simulink subsystem "Vehicle"  (R2023b)
settings: Solver=VariableStepAuto  StartTime=0.0  StopTime=10.0  RelTol=1e-3
undefined symbols (not defined in the file): Earth, WGS84
libraries: aerolibtransform2 x1
settings Model: Creator=szdaniel  LastModifiedBy=szdaniel

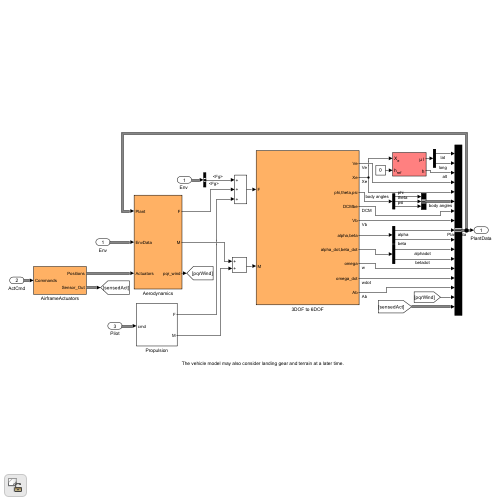
[thumbnail: Simulink's stored preview of the top-level diagram]
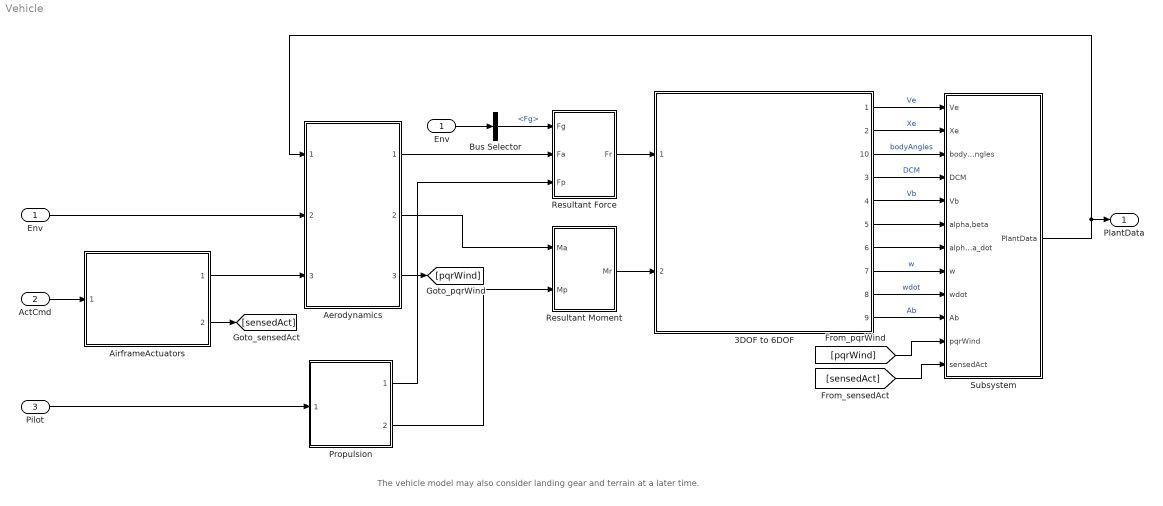
== system Vehicle ==
  note: The vehicle model may also consider landing gear and terrain at a later time.
  Env : Inport
  ActCmd : Inport  Port=2  OutDataTypeStr=Bus: ActuatorCmdBus
  Pilot : Inport  Port=3  OutDataTypeStr=Bus: PilotCmdBus
  3DOF to 6DOF : Subsystem  ReferencedSubsystem=s3DOF_to_6DOF
      settings: PortSchema="{\"entries\":[{\"content\":{\"sides\":[{\"content\":{\"connectorIds\":[\"In1\",\"In2\"]},\"type\":\"ConnectorPlacement.EquallySpacedRectSide\",\"uuid\":\"ca33f1ca-0408-408f-8b83-1949eaea45ca\"},{\"content\":{\"connectorIds\":[\"Out1\",\"Out2\",\"Out10\",\"Out3\",\"Out4\",\"Out5\",\"Out6\",\"Out7\",\"Out8\",\"Out9\"],\"side\":\"RIGHT\"},\"type\":\"ConnectorPlacement.EquallySpacedRectSide\",\"uuid\":\"ad7e90e7-3dbe-47fd-95f1-532738b13a23\"},{\"content\":{\"side\":\"TOP\"},\"type\":\"ConnectorPlacement.EquallySpacedRectSide\",\"uuid\":\"eb3caa52-9404-4bf8-ba4e-b768e3179a3f\"}]},\"type\":\"ConnectorPlacement.EquallySpacedConnector\",\"uuid\":\"d12b1c57-6f02-4c3c-8b19-49af329e35c6\"}],\"packageUris\":[\"http://schema.mathworks.com/mf0/Connector/R2020b\"],\"version\":\"1.0\"}"
  Aerodynamics : Subsystem  ReferencedSubsystem=Aerodynamics
  AirframeActuators : Subsystem  ReferencedSubsystem=AirframeActuators
  Bus Selector : BusSelector  OutputSignals=Fg
  "Env " : InportShadow
  Propulsion : Subsystem  ReferencedSubsystem=Propulsion
      settings: RTWSystemCode=Inline
  Resultant Force : Subsystem
  Resultant Moment : Subsystem
  Subsystem : Subsystem
  PlantData : Outport  VectorParamsAs1DForOutWhenUnconnected=off
  wires:
  Env/1 -> Aerodynamics/2
  ActCmd/1 -> AirframeActuators/1
  Pilot/1 -> Propulsion/1
  AirframeActuators/1 -> Aerodynamics/3
  Aerodynamics/3 -> [pqrWind]
  AirframeActuators/2 -> [sensedAct]
  Aerodynamics/2 -> Resultant Moment/1(Ma)
  Propulsion/2 -> Resultant Moment/2(Mp)
  Resultant Moment/1(Mr) -> 3DOF to 6DOF/2
  "Env "/1 -> Bus Selector/1
  Aerodynamics/1 -> Resultant Force/2(Fa)
  Propulsion/1 -> Resultant Force/3(Fp)
  Resultant Force/1(Fr) -> 3DOF to 6DOF/1
  Bus Selector/1 -> Resultant Force/1(Fg)  "<Fg>"
  Subsystem/1(PlantData) -> PlantData/1, Aerodynamics/1
  3DOF to 6DOF/1 -> Subsystem/1(Ve)  "Ve"
  3DOF to 6DOF/2 -> Subsystem/2(Xe)  "Xe"
  3DOF to 6DOF/10 -> Subsystem/3(bodyAngles)  "bodyAngles"
  3DOF to 6DOF/3 -> Subsystem/4(DCM)  "DCM"
  3DOF to 6DOF/4 -> Subsystem/5(Vb)  "Vb"
  3DOF to 6DOF/5 -> Subsystem/6(alpha,beta)
  3DOF to 6DOF/6 -> Subsystem/7(alpha_dot,beta_dot)
  3DOF to 6DOF/7 -> Subsystem/8(w)  "w"
  3DOF to 6DOF/8 -> Subsystem/9(wdot)  "wdot"
  3DOF to 6DOF/9 -> Subsystem/10(Ab)  "Ab"
  [pqrWind] -> Subsystem/11(pqrWind)
  [sensedAct] -> Subsystem/12(sensedAct)

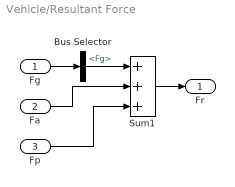
== system Vehicle/Resultant Force ==
  Fg : Inport
  Fa : Inport  Port=2
  Fp : Inport  Port=3
  Bus Selector : BusSelector  OutputSignals=Fg
  Sum1 : Sum  Inputs=+++  InputSameDT=on  SaturateOnIntegerOverflow=on  OutDataTypeStr=Inherit: Same as first input
  Fr : Outport
  wires:
  Sum1/1 -> Fr/1
  Fa/1 -> Sum1/2
  Bus Selector/1 -> Sum1/1  "<Fg>"
  Fg/1 -> Bus Selector/1
  Fp/1 -> Sum1/3

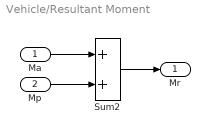
== system Vehicle/Resultant Moment ==
  Ma : Inport
  Mp : Inport  Port=2
  Sum2 : Sum  InputSameDT=on  SaturateOnIntegerOverflow=on  OutDataTypeStr=Inherit: Same as first input
  Mr : Outport
  wires:
  Sum2/1 -> Mr/1
  Ma/1 -> Sum2/1
  Mp/1 -> Sum2/2

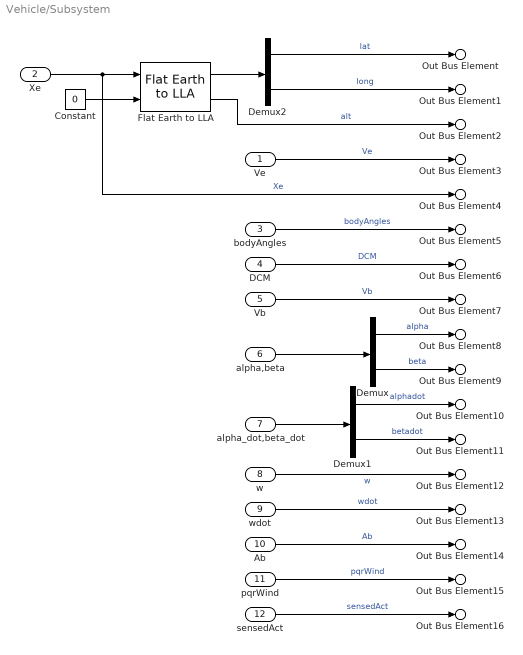
== system Vehicle/Subsystem ==
  Ve : Inport
  Xe : Inport  Port=2
  bodyAngles : Inport  Port=3
  DCM : Inport  Port=4
  Vb : Inport  Port=5
  alpha,beta : Inport  Port=6
  alpha_dot,beta_dot : Inport  Port=7
  w : Inport  Port=8
  wdot : Inport  Port=9
  Ab : Inport  Port=10
  pqrWind : Inport  Port=11
  sensedAct : Inport  Port=12
  Constant : Constant  Value=0
  Demux : Demux  Outputs=2
  Demux1 : Demux  Outputs=2
  Demux2 : Demux  Outputs=2
  Flat Earth to LLA : aerolibtransform2/Flat Earth to LLA  units=Metric (MKS)  ptype=Earth (WGS84)  F=1/298.257223563  R=6378137  refPosPort=off  LL0=LatLong0  psi=heading0
  Out Bus Element : Outport  PortName=PlantData  Element=lat
  Out Bus Element1 : Outport  PortName=PlantData  Element=lon
  Out Bus Element2 : Outport  PortName=PlantData  Element=alt
  Out Bus Element3 : Outport  PortName=PlantData  Element=Ve
  Out Bus Element4 : Outport  PortName=PlantData  Element=Xe
  Out Bus Element5 : Outport  PortName=PlantData  Element=bodyAngles
  Out Bus Element6 : Outport  PortName=PlantData  Element=DCM
  Out Bus Element7 : Outport  PortName=PlantData  Element=Vb
  Out Bus Element8 : Outport  PortName=PlantData  Element=alpha
  Out Bus Element9 : Outport  PortName=PlantData  Element=beta
  Out Bus Element10 : Outport  PortName=PlantData  Element=alphadot
  Out Bus Element11 : Outport  PortName=PlantData  Element=betadot
  Out Bus Element12 : Outport  PortName=PlantData  Element=w
  Out Bus Element13 : Outport  PortName=PlantData  Element=wdot
  Out Bus Element14 : Outport  PortName=PlantData  Element=Ab
  Out Bus Element15 : Outport  PortName=PlantData  Element=WindAngularRates
  Out Bus Element16 : Outport  PortName=PlantData  Element=ActPositions
  wires:
  pqrWind/1 -> Out Bus Element15/1  "pqrWind"
  sensedAct/1 -> Out Bus Element16/1  "sensedAct"
  Ab/1 -> Out Bus Element14/1  "Ab"
  w/1 -> Out Bus Element12/1  "w"
  wdot/1 -> Out Bus Element13/1  "wdot"
  Demux1/1 -> Out Bus Element10/1  "alphadot"
  DCM/1 -> Out Bus Element6/1  "DCM"
  Vb/1 -> Out Bus Element7/1  "Vb"
  Ve/1 -> Out Bus Element3/1  "Ve"
  alpha_dot,beta_dot/1 -> Demux1/1
  alpha,beta/1 -> Demux/1
  Demux2/1 -> Out Bus Element/1  "lat"
  Demux1/2 -> Out Bus Element11/1  "betadot"
  Constant/1 -> Flat Earth to LLA/2
  Flat Earth to LLA/2 -> Out Bus Element2/1  "alt"
  Flat Earth to LLA/1 -> Demux2/1
  Demux2/2 -> Out Bus Element1/1  "long"
  Xe/1 -> Flat Earth to LLA/1, Out Bus Element4/1  "Xe"
  bodyAngles/1 -> Out Bus Element5/1  "bodyAngles"
  Demux/1 -> Out Bus Element8/1  "alpha"
  Demux/2 -> Out Bus Element9/1  "beta"
